simulink model "ModeInputHandle"  (R2018b)
settings: Solver=FixedStepDiscrete  StartTime=0.0  StopTime=10.0  FixedStep=0.01  RelTol=1e-3
undefined symbols (not defined in the file or in its folder): c, CmprtMdHMIReqExt2Tp1, CmprtMdHMIReqExtTp1, CmprtMdHMIReqTp1, d, e, EZESwReq1, f, g, IfVeSMSeStNumConfig, j, KeSMSuButtonLongPressedThrshldTm_Val, KeSMSuFoldType_Val, KeSMSwSeatSMSSeatMdTrigGapTimer_Val, KeSMSwSeatTrigWaitTimer_Val, KeSMSwSRSActiveValidTm_Val, LckUlckActvtFunc1, LstLckFunc1, LugSelectSw1, MdReqTp1, PowerMode1, SeatOccupiedSts1, SRSMode1, StPassCmprtMdCtrl_Md10_VCUConfig_Val, StPassCmprtMdCtrl_Md11_VCUConfig_Val, StPassCmprtMdCtrl_Md12_VCUConfig_Val, StPassCmprtMdCtrl_Md13_VCUConfig_Val, StPassCmprtMdCtrl_Md1_VCUConfig_Val, StPassCmprtMdCtrl_Md27_VCUConfig_Val, StPassCmprtMdCtrl_Md28_VCUConfig_Val, StPassCmprtMdCtrl_Md29_VCUConfig_Val, StPassCmprtMdCtrl_Md2_VCUConfig_Val, StPassCmprtMdCtrl_Md30_VCUConfig_Val, StPassCmprtMdCtrl_Md31_VCUConfig_Val, StPassCmprtMdCtrl_Md32_VCUConfig_Val, StPassCmprtMdCtrl_Md3_VCUConfig_Val, StPassCmprtMdCtrl_Md53_VCUConfig_Val, StPassCmprtMdCtrl_Md56_VCUConfig_Val, StPassCmprtMdCtrl_Md57_VCUConfig_Val, StPassCmprtMdCtrl_Md58_VCUConfig_Val, StPassCmprtMdCtrl_Md61_VCUConfig_Val, StPassCmprtMdCtrl_Md62_VCUConfig_Val, StPassCmprtMdCtrl_Md8_VCUConfig_Val, StPassCmprtMdCtrl_Md9_VCUConfig_Val, StSrv_StMd10_Config_Val, StSrv_StMd11_Config_Val, StSrv_StMd12_Config_Val, StSrv_StMd13_Config_Val, StSrv_StMd1_Config_Val, StSrv_StMd27_Config_Val, StSrv_StMd28_Config_Val, StSrv_StMd29_Config_Val, StSrv_StMd2_Config_Val, StSrv_StMd30_Config_Val, StSrv_StMd31_Config_Val, StSrv_StMd32_Config_Val, StSrv_StMd3_Config_Val, StSrv_StMd8_Config_Val, StSrv_StMd9_Config_Val, VehMovState1
libraries: MSMLib x91
(part 3 of 9)

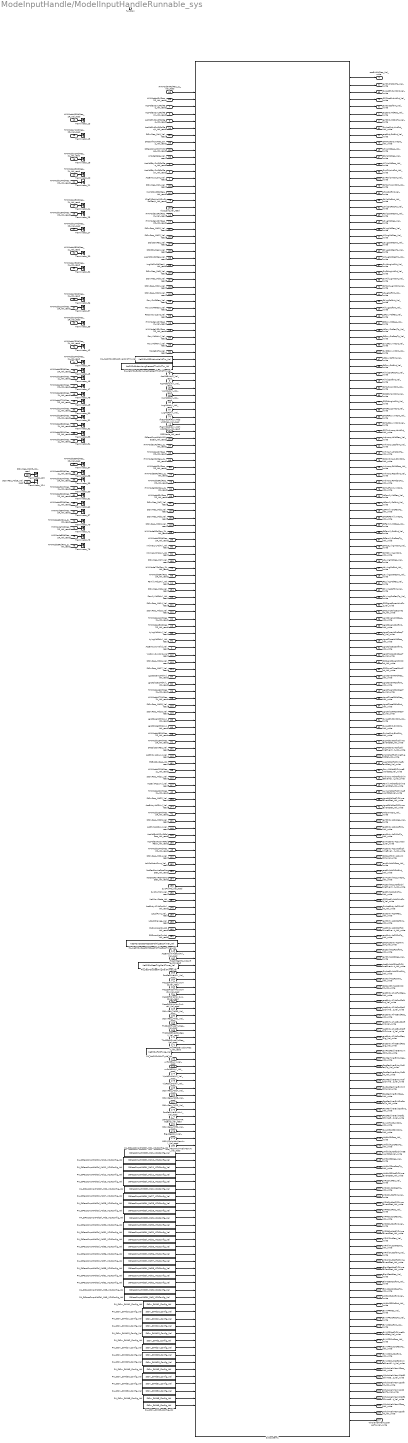
== system ModeInputHandle/ModelInputHandleRunnable_sys ==
  AcsEntry2LSwt_Val_read : Inport
  AcsEntrySwValid_Val_read : Inport  Port=2
  AcsMdEntyAvl_Val_read : Inport  Port=3
  AcsMdEtrySwRtRclReq_Val_read : Inport  Port=4
  AcsMdEtrySwRtRclReqV_Val_read : Inport  Port=5
  AcsMdExtAvl_Val_read : Inport  Port=6
  AcsMdExtSwLtRclReq_Val_read : Inport  Port=7
  AcsMdExtSwLtRclReqV_Val_read : Inport  Port=8
  AcsMdExtSwRtRclReq_Val_read : Inport  Port=9
  AcsMdExtSwRtRclReqV_Val_read : Inport  Port=10
  FamilyMdLtAvl_Val_read : Inport  Port=11
  FamilyMdRtAvl_Val_read : Inport  Port=12
  HMIMode10RclReq_2R_Val_read : Inport  Port=13
  HMIMode10RclReq_2L_Val_read : Inport  Port=14
  HMIMode11RclReq_2R_Val_read : Inport  Port=15
  HMIMode11RclReq_2L_Val_read : Inport  Port=16
  HMIMode12RclReq_2R_Val_read : Inport  Port=17
  HMIMode12RclReq_2L_Val_read : Inport  Port=18
  HMIMode13RclReq_2R_Val_read : Inport  Port=19
  HMIMode13RclReq_2L_Val_read : Inport  Port=20
  HMIMode14RclReq_2R_Val_read : Inport  Port=21
  HMIMode14RclReq_2L_Val_read : Inport  Port=22
  HMIMode15RclReq_2R_Val_read : Inport  Port=23
  HMIMode15RclReq_2L_Val_read : Inport  Port=24
  HMIMode16RclReq_2R_Val_read : Inport  Port=25
  HMIMode16RclReq_2L_Val_read : Inport  Port=26
  HMIMode17RclReq_2R_Val_read : Inport  Port=27
  HMIMode17RclReq_2L_Val_read : Inport  Port=28
  HMIMode18RclReq_2R_Val_read : Inport  Port=29
  HMIMode18RclReq_2L_Val_read : Inport  Port=30
  HMIMode19RclReq_2R_Val_read : Inport  Port=31
  HMIMode19RclReq_2L_Val_read : Inport  Port=32
  HMIMode1RclReq_2R_Val_read : Inport  Port=33
  HMIMode1RclReq_2L_Val_read : Inport  Port=34
  HMIMode20RclReq_2R_Val_read : Inport  Port=35
  HMIMode20RclReq_2L_Val_read : Inport  Port=36
  HMIMode21RclReq_2R_Val_read : Inport  Port=37
  HMIMode21RclReq_2L_Val_read : Inport  Port=38
  HMIMode22RclReq_2R_Val_read : Inport  Port=39
  HMIMode22RclReq_2L_Val_read : Inport  Port=40
  HMIMode23RclReq_2R_Val_read : Inport  Port=41
  HMIMode23RclReq_2L_Val_read : Inport  Port=42
  HMIMode24RclReq_2R_Val_read : Inport  Port=43
  HMIMode24RclReq_2L_Val_read : Inport  Port=44
  HMIMode25RclReq_2R_Val_read : Inport  Port=45
  HMIMode25RclReq_2L_Val_read : Inport  Port=46
  HMIMode26RclReq_2R_Val_read : Inport  Port=47
  HMIMode26RclReq_2L_Val_read : Inport  Port=48
  HMIMode27RclReq_2R_Val_read : Inport  Port=49
  HMIMode27RclReq_2L_Val_read : Inport  Port=50
  HMIMode28RclReq_2R_Val_read : Inport  Port=51
  HMIMode28RclReq_2L_Val_read : Inport  Port=52
  HMIMode29RclReq_2R_Val_read : Inport  Port=53
  HMIMode29RclReq_2L_Val_read : Inport  Port=54
  HMIMode2RclReq_2R_Val_read : Inport  Port=55
  HMIMode2RclReq_2L_Val_read : Inport  Port=56
  HMIMode30RclReq_2R_Val_read : Inport  Port=57
  HMIMode30RclReq_2L_Val_read : Inport  Port=58
  HMIMode31RclReq_2R_Val_read : Inport  Port=59
  HMIMode31RclReq_2L_Val_read : Inport  Port=60
  HMIMode32RclReq_2R_Val_read : Inport  Port=61
  HMIMode32RclReq_2L_Val_read : Inport  Port=62
  HMIMode3RclReq_2R_Val_read : Inport  Port=63
  HMIMode3RclReq_2L_Val_read : Inport  Port=64
  HMIMode4RclReq_2R_Val_read : Inport  Port=65
  HMIMode4RclReq_2L_Val_read : Inport  Port=66
  HMIMode5RclReq_2R_Val_read : Inport  Port=67
  HMIMode5RclReq_2L_Val_read : Inport  Port=68
  HMIMode6RclReq_2R_Val_read : Inport  Port=69
  HMIMode6RclReq_2L_Val_read : Inport  Port=70
  HMIMode7RclReq_2R_Val_read : Inport  Port=71
  HMIMode7RclReq_2L_Val_read : Inport  Port=72
  HMIMode8RclReq_2R_Val_read : Inport  Port=73
  HMIMode8RclReq_2L_Val_read : Inport  Port=74
  HMIMode9RclReq_2R_Val_read : Inport  Port=75
  HMIMode9RclReq_2L_Val_read : Inport  Port=76
  IfVeSMSbRrRcvyMdSwRclReq_Val_read : Inport  Port=77
  IfVeSMSbRrRcvyMdSwRclReqV_Val_read : Inport  Port=78
  IfVeSMSeVipMdSwRtRclReqV_Val_read : Inport  Port=79
  IntimacyLMdAvl_Val_read : Inport  Port=80
  IntimacyRMdAvl_Val_read : Inport  Port=81
  LgrstCloseLtMdAvl_Val_read : Inport  Port=82
  LgrstCloseRtMdAvl_Val_read : Inport  Port=83
  LgrstOpenLtMdAvl_Val_read : Inport  Port=84
  LgrstOpenRtMdAvl_Val_read : Inport  Port=85
  LugMdLtAvl_Val_read : Inport  Port=86
  LugMdRtAvl_Val_read : Inport  Port=87
  LugMdSwRclReq_Val_read : Inport  Port=88
  LugMdSwRclReqV_Val_read : Inport  Port=89
  LyingMdLtAvl_Val_read : Inport  Port=90
  LyingMdRtAvl_Val_read : Inport  Port=91
  ModeSrcTp_Val_read : Inport  Port=92
  oModeState_Val_read : Inport  Port=93
  RcvyMdLtAvl_Val_read : Inport  Port=94
  RcvyMdRtAvl_Val_read : Inport  Port=95
  RcvySwRtReq_Val_read : Inport  Port=96
  RcvySwRtReqV_Val_read : Inport  Port=97
  Recovery2LSwt_Val_read : Inport  Port=98
  SRSCnfmSwReq_67_2_Val_read : Inport  Port=99
  SRSMode_Val_read : Inport  Port=100
  SRSSlctSwReq_Val_read : Inport  Port=101
  StPassCmprtMdHMIReq_Val_read : Inport  Port=102
  StPassCmprtMdHMIReqExt_Val_read : Inport  Port=103
  StSlctSwReq_Val_read : Inport  Port=104
  StSlctSwReqV_Val_read : Inport  Port=105
  StSrvReq_Md1_Val_read : Inport  Port=106
  StSrvReq_Md10_Val_read : Inport  Port=107
  StSrvReq_Md11_Val_read : Inport  Port=108
  StSrvReq_Md12_Val_read : Inport  Port=109
  StSrvReq_Md13_Val_read : Inport  Port=110
  StSrvReq_Md14_Val_read : Inport  Port=111
  StSrvReq_Md15_Val_read : Inport  Port=112
  StSrvReq_Md16_Val_read : Inport  Port=113
  StSrvReq_Md17_Val_read : Inport  Port=114
  StSrvReq_Md18_Val_read : Inport  Port=115
  StSrvReq_Md19_Val_read : Inport  Port=116
  StSrvReq_Md2_Val_read : Inport  Port=117
  StSrvReq_Md20_Val_read : Inport  Port=118
  StSrvReq_Md21_Val_read : Inport  Port=119
  StSrvReq_Md22_Val_read : Inport  Port=120
  StSrvReq_Md23_Val_read : Inport  Port=121
  StSrvReq_Md24_Val_read : Inport  Port=122
  StSrvReq_Md25_Val_read : Inport  Port=123
  StSrvReq_Md26_Val_read : Inport  Port=124
  StSrvReq_Md27_Val_read : Inport  Port=125
  StSrvReq_Md28_Val_read : Inport  Port=126
  StSrvReq_Md29_Val_read : Inport  Port=127
  StSrvReq_Md3_Val_read : Inport  Port=128
  StSrvReq_Md30_Val_read : Inport  Port=129
  StSrvReq_Md31_Val_read : Inport  Port=130
  StSrvReq_Md32_Val_read : Inport  Port=131
  StSrvReq_Md4_Val_read : Inport  Port=132
  StSrvReq_Md5_Val_read : Inport  Port=133
  StSrvReq_Md6_Val_read : Inport  Port=134
  StSrvReq_Md7_Val_read : Inport  Port=135
  StSrvReq_Md8_Val_read : Inport  Port=136
  StSrvReq_Md9_Val_read : Inport  Port=137
  Vip2LSwt_Val_read : Inport  Port=138
  VipMdLtAvl_Val_read : Inport  Port=139
  VipMdRtAvl_Val_read : Inport  Port=140
  VipMdSwRtRclReq_Val_read : Inport  Port=141
  VipRcvySwValid_Val_read : Inport  Port=142
  AcsEntry4s2LAvl_Val_read : Inport  Port=143
  AcsEntry4s2RAvl_Val_read : Inport  Port=144
  AcsEntryAll4sBwdAvl_Val_read : Inport  Port=145
  AcsEntryAll4sFwdAvl_Val_read : Inport  Port=146
  AcsExit4s2LAvl_Val_read : Inport  Port=147
  AcsExit4s2RAvl_Val_read : Inport  Port=148
  AcsMdExt4SSwRtRclReq_Val_read : Inport  Port=149
  AcsMdExt4SSwRtRclReqV_Val_read : Inport  Port=150
  EZE4SSwReq_Val_read : Inport  Port=151
  LckUlckActvtFunc_Val_read : Inport  Port=152
  NotSecRowLeSeaOccStat_Val_read : Inport  Port=153
  NotSecRowRtSeaOccStat_Val_read : Inport  Port=154
  SysPwrMd_Val_read : Inport  Port=155
  SysPwrMdV_Val_read : Inport  Port=156
  VehMovState_Val_read : Inport  Port=157
  LstLckChange_Val_read : Inport  Port=158
  LstLckFunc_Val_read : Inport  Port=159
  RLDoorAjarSwAct_Val_read : Inport  Port=160
  RRDoorAjarSwAct_Val_read : Inport  Port=161
  IfVeSMSeStNumConfig_Val_read : Inport  Port=162
  PasReclinerAvl_Val_read : Inport  Port=163
  PassStFldDnMovSwAct_Val_read : Inport  Port=164
  PassStFldDnMovSwActV_Val_read : Inport  Port=165
  PassStFldUpMovSwAct_Val_read : Inport  Port=166
  PassStFldUpMovSwActV_Val_read : Inport  Port=167
  ThdRLtStExpdSwReq_Val_read : Inport  Port=168
  ThdRLtStExpdSwReqV_Val_read : Inport  Port=169
  ThdRRtStExpdSwReq_Val_read : Inport  Port=170
  ThdRRtStExpdSwReqV_Val_read : Inport  Port=171
  unfold3LAvl_Val_read : Inport  Port=172
  unfold3RAvl_Val_read : Inport  Port=173
  VipLtOutMdAvl_Val_read : Inport  Port=174
  VipRtOutMdAvl_Val_read : Inport  Port=175
  PasReclinerExitAvl_Val_read : Inport  Port=176
  StPassCmprtMdHMIReqExt2_Val_read : Inport  Port=177
  Big4SeatAvl_Val_read : Inport  Port=178
  M61WholeVehMemAvl_Val_read : Inport  Port=179
  M62WholeVehMemAvl_Val_read : Inport  Port=180
  function : TriggerPort  TriggerType=function-call  VariantControl=(inherit)  SampleTimeType=periodic  SampleTime=-1
  PA_KeSMSuButtonLongPressedThrshldTm_Val : Constant  Value=KeSMSuButtonLongPressedThrshldTm_Val
  PA_KeSMSuFoldType_Val : Constant  Value=KeSMSuFoldType_Val
  PA_KeSMSwSRSActiveValidTm_Val : Constant  Value=KeSMSwSRSActiveValidTm_Val
  PA_KeSMSwSeatSMSSeatMdTrigGapTimer_Val : Constant  Value=KeSMSwSeatSMSSeatMdTrigGapTimer_Val
  PA_KeSMSwSeatTrigWaitTimer_Val : Constant  Value=KeSMSwSeatTrigWaitTimer_Val
  PA_StPassCmprtMdCtrl_Md10_VCUConfig_Val : Constant  Value=StPassCmprtMdCtrl_Md10_VCUConfig_Val
  PA_StPassCmprtMdCtrl_Md11_VCUConfig_Val : Constant  Value=StPassCmprtMdCtrl_Md11_VCUConfig_Val
  PA_StPassCmprtMdCtrl_Md12_VCUConfig_Val : Constant  Value=StPassCmprtMdCtrl_Md12_VCUConfig_Val
  PA_StPassCmprtMdCtrl_Md13_VCUConfig_Val : Constant  Value=StPassCmprtMdCtrl_Md13_VCUConfig_Val
  PA_StPassCmprtMdCtrl_Md1_VCUConfig_Val : Constant  Value=StPassCmprtMdCtrl_Md1_VCUConfig_Val
  PA_StPassCmprtMdCtrl_Md27_VCUConfig_Val : Constant  Value=StPassCmprtMdCtrl_Md27_VCUConfig_Val
  PA_StPassCmprtMdCtrl_Md28_VCUConfig_Val : Constant  Value=StPassCmprtMdCtrl_Md28_VCUConfig_Val
  PA_StPassCmprtMdCtrl_Md29_VCUConfig_Val : Constant  Value=StPassCmprtMdCtrl_Md29_VCUConfig_Val
  PA_StPassCmprtMdCtrl_Md2_VCUConfig_Val : Constant  Value=StPassCmprtMdCtrl_Md2_VCUConfig_Val
  PA_StPassCmprtMdCtrl_Md30_VCUConfig_Val : Constant  Value=StPassCmprtMdCtrl_Md30_VCUConfig_Val
  PA_StPassCmprtMdCtrl_Md31_VCUConfig_Val : Constant  Value=StPassCmprtMdCtrl_Md31_VCUConfig_Val
  PA_StPassCmprtMdCtrl_Md32_VCUConfig_Val : Constant  Value=StPassCmprtMdCtrl_Md32_VCUConfig_Val
  PA_StPassCmprtMdCtrl_Md3_VCUConfig_Val : Constant  Value=StPassCmprtMdCtrl_Md3_VCUConfig_Val
  PA_StPassCmprtMdCtrl_Md53_VCUConfig_Val : Constant  Value=StPassCmprtMdCtrl_Md53_VCUConfig_Val
  PA_StPassCmprtMdCtrl_Md56_VCUConfig_Val : Constant  Value=StPassCmprtMdCtrl_Md56_VCUConfig_Val
  PA_StPassCmprtMdCtrl_Md57_VCUConfig_Val : Constant  Value=StPassCmprtMdCtrl_Md57_VCUConfig_Val
  PA_StPassCmprtMdCtrl_Md58_VCUConfig_Val : Constant  Value=StPassCmprtMdCtrl_Md58_VCUConfig_Val
  PA_StPassCmprtMdCtrl_Md61_VCUConfig_Val : Constant  Value=StPassCmprtMdCtrl_Md61_VCUConfig_Val
  PA_StPassCmprtMdCtrl_Md62_VCUConfig_Val : Constant  Value=StPassCmprtMdCtrl_Md62_VCUConfig_Val
  PA_StPassCmprtMdCtrl_Md8_VCUConfig_Val : Constant  Value=StPassCmprtMdCtrl_Md8_VCUConfig_Val
  PA_StPassCmprtMdCtrl_Md9_VCUConfig_Val : Constant  Value=StPassCmprtMdCtrl_Md9_VCUConfig_Val
  PA_StSrv_StMd10_Config_Val : Constant  Value=StSrv_StMd10_Config_Val
  PA_StSrv_StMd11_Config_Val : Constant  Value=StSrv_StMd11_Config_Val
  PA_StSrv_StMd12_Config_Val : Constant  Value=StSrv_StMd12_Config_Val
  PA_StSrv_StMd13_Config_Val : Constant  Value=StSrv_StMd13_Config_Val
  PA_StSrv_StMd1_Config_Val : Constant  Value=StSrv_StMd1_Config_Val
  PA_StSrv_StMd27_Config_Val : Constant  Value=StSrv_StMd27_Config_Val
  PA_StSrv_StMd28_Config_Val : Constant  Value=StSrv_StMd28_Config_Val
  PA_StSrv_StMd29_Config_Val : Constant  Value=StSrv_StMd29_Config_Val
  PA_StSrv_StMd2_Config_Val : Constant  Value=StSrv_StMd2_Config_Val
  PA_StSrv_StMd30_Config_Val : Constant  Value=StSrv_StMd30_Config_Val
  PA_StSrv_StMd31_Config_Val : Constant  Value=StSrv_StMd31_Config_Val
  PA_StSrv_StMd32_Config_Val : Constant  Value=StSrv_StMd32_Config_Val
  PA_StSrv_StMd3_Config_Val : Constant  Value=StSrv_StMd3_Config_Val
  PA_StSrv_StMd8_Config_Val : Constant  Value=StSrv_StMd8_Config_Val
  PA_StSrv_StMd9_Config_Val : Constant  Value=StSrv_StMd9_Config_Val
  Subsystem1 : Subsystem
  Terminator_{13,15,18,20..21,24..25,27,30,32,36..37,39,42,44..54,57..62,67,70..71,73,76,123..124} (38 alike) : Terminator
  acsEntyMdReq_Val_write : Outport
  acsEntyMdSrcTp_Val_write : Outport  Port=2
  acsEntySoftInt_Val_write : Outport  Port=3
  acsExtMdReq_Val_write : Outport  Port=4
  acsExtMdSrcTp_Val_write : Outport  Port=5
  acsExtSoftInt_Val_write : Outport  Port=6
  acsMdEntryNotf1ChimeEventStat_Val_write : Outport  Port=7
  acsMdExtNotf1ChimeEventStat_Val_write : Outport  Port=8
  AllLugMdReq_Val_write : Outport  Port=9
  AllLugSoftInt_Val_write : Outport  Port=10
  AllLugSrcReqTp_Val_write : Outport  Port=11
  AllVipMdReq_Val_write : Outport  Port=12
  AllVipSoftInt_Val_write : Outport  Port=13
  AllVipSrcReqTp_Val_write : Outport  Port=14
  FamilyMdNotf1ChimeEventStat_Val_write : Outport  Port=15
  IntimacyMdNotf1ChimeEventStat_Val_write : Outport  Port=16
  IntimacyLtMdReq_Val_write : Outport  Port=17
  IntimacyLtMdSrcTp_Val_write : Outport  Port=18
  IntimacyRtMdReq_Val_write : Outport  Port=19
  IntimacyRtMdSrcTp_Val_write : Outport  Port=20
  IntimacyRtSoftInt_Val_write : Outport  Port=21
  IntimacyLtSoftInt_Val_write : Outport  Port=22
  LtFamilyMdReq_Val_write : Outport  Port=23
  LtFamilySoftInt_Val_write : Outport  Port=24
  LtFamilySrcReqTp_Val_write : Outport  Port=25
  LtLyingMdReq_Val_write : Outport  Port=26
  LtLyingSoftInt_Val_write : Outport  Port=27
  LtLyingSrcReqTp_Val_write : Outport  Port=28
  LgrstCloseLtMdReq_Val_write : Outport  Port=29
  LgrstCloseLtSrcReqTp_Val_write : Outport  Port=30
  LgrstCloseLtSoftInt_Val_write : Outport  Port=31
  LgrstCloseRtMdReq_Val_write : Outport  Port=32
  LgrstCloseRtSrcReqTp_Val_write : Outport  Port=33
  LgrstCloseRtSoftInt_Val_write : Outport  Port=34
  LgrstLtMdNotf1ChimeEventStat_Val_write : Outport  Port=35
  LgrstOpenLtMdReq_Val_write : Outport  Port=36
  LgrstOpenLtSrcReqTp_Val_write : Outport  Port=37
  LgrstOpenLtSoftInt_Val_write : Outport  Port=38
  LgrstOpenRtMdReq_Val_write : Outport  Port=39
  LgrstOpenRtSrcReqTp_Val_write : Outport  Port=40
  LgrstOpenRtSoftInt_Val_write : Outport  Port=41
  LgrstRtMdNotf1ChimeEventStat_Val_write : Outport  Port=42
  LtLugMdReq_Val_write : Outport  Port=43
  LtLugSoftInt_Val_write : Outport  Port=44
  LtLugSrcReqTp_Val_write : Outport  Port=45
  LtRcvyMdReq_Val_write : Outport  Port=46
  LtRcvySoftInt_Val_write : Outport  Port=47
  LtRcvySrcReqTp_Val_write : Outport  Port=48
  LtVipMdReq_Val_write : Outport  Port=49
  LtVipSoftInt_Val_write : Outport  Port=50
  LtVipSrcReqTp_Val_write : Outport  Port=51
  LugMdNotf1ChimeEventStat_Val_write : Outport  Port=52
  LyingMdNotf1ChimeEventStat_Val_write : Outport  Port=53
  RcvyMdNotf1ChimeEventStat_Val_write : Outport  Port=54
  RtFamilyMdReq_Val_write : Outport  Port=55
  RtFamilySoftInt_Val_write : Outport  Port=56
  RtFamilySrcReqTp_Val_write : Outport  Port=57
  RtLugMdReq_Val_write : Outport  Port=58
  RtLugSoftInt_Val_write : Outport  Port=59
  RtLugSrcReqTp_Val_write : Outport  Port=60
  RtLyingMdReq_Val_write : Outport  Port=61
  RtLyingSoftInt_Val_write : Outport  Port=62
  RtLyingSrcReqTp_Val_write : Outport  Port=63
  RtRcvyMdReq_Val_write : Outport  Port=64
  RtRcvySoftInt_Val_write : Outport  Port=65
  RtRcvySrcReqTp_Val_write : Outport  Port=66
  RtVipMdReq_Val_write : Outport  Port=67
  RtVipSoftInt_Val_write : Outport  Port=68
  RtVipSrcReqTp_Val_write : Outport  Port=69
  SRSAcsEntyIntCnt_Val_write : Outport  Port=70
  SRSAcsExtIntCnt_Val_write : Outport  Port=71
  SRSAllLugIntCnt_Val_write : Outport  Port=72
  SRSAllVipIntCnt_Val_write : Outport  Port=73
  SRSIntimacyLtIntCnt_Val_write : Outport  Port=74
  SRSIntimacyRtIntCnt_Val_write : Outport  Port=75
  SRSLtFamilyIntCnt_Val_write : Outport  Port=76
  SRSLtLugIntCnt_Val_write : Outport  Port=77
  SRSLtLyingIntCnt_Val_write : Outport  Port=78
  SRSLtRcvyIntCnt_Val_write : Outport  Port=79
  SRSLtVipIntCnt_Val_write : Outport  Port=80
  SRSLgrstCloseLtIntCnt_Val_write : Outport  Port=81
  SRSLgrstCloseRtIntCnt_Val_write : Outport  Port=82
  SRSLgrstOpenLtIntCnt_Val_write : Outport  Port=83
  SRSLgrstOpenRtIntCnt_Val_write : Outport  Port=84
  SRSRtFamilyIntCnt_Val_write : Outport  Port=85
  SRSRtLugIntCnt_Val_write : Outport  Port=86
  SRSRtLyingIntCnt_Val_write : Outport  Port=87
  SRSRtRcvyIntCnt_Val_write : Outport  Port=88
  SRSRtVipIntCnt_Val_write : Outport  Port=89
  SwAcsEntyBIntCnt_Val_write : Outport  Port=90
  SwAcsEntyLIntCnt_Val_write : Outport  Port=91
  SwAcsEntyRIntCnt_Val_write : Outport  Port=92
  SwAcsExtLIntCnt_Val_write : Outport  Port=93
  SwAcsExtRIntCnt_Val_write : Outport  Port=94
  SwAllLugIntCnt_Val_write : Outport  Port=95
  SwLfVipIntCnt_Val_write : Outport  Port=96
  SwLtLugIntCnt_Val_write : Outport  Port=97
  SwLtRcvyIntCnt_Val_write : Outport  Port=98
  SwRtLugIntCnt_Val_write : Outport  Port=99
  SwRtRcvyIntCnt_Val_write : Outport  Port=100
  SwRtVipIntCnt_Val_write : Outport  Port=101
  VipMdNotf1ChimeEventStat_Val_write : Outport  Port=102
  MdSWIntSrc_Val_write : Outport  Port=103
  SwAcsEntry4s2LIntCnt_Val_write : Outport  Port=104
  AcsEntry4s2LNotf1ChimeEventStat_Val_write : Outport  Port=105
  acsEntry4s2LReq_Val_write : Outport  Port=106
  acsEntry4s2LSoftInt_Val_write : Outport  Port=107
  acsEntry4s2LSrcTp_Val_write : Outport  Port=108
  SwAcsEntry4s2RIntCnt_Val_write : Outport  Port=109
  AcsEntry4s2RNotf1ChimeEventStat_Val_write : Outport  Port=110
  acsEntry4s2RReq_Val_write : Outport  Port=111
  acsEntry4s2RSoftInt_Val_write : Outport  Port=112
  acsEntry4s2RSrcTp_Val_write : Outport  Port=113
  AcsEntryAll4sBwdNotf1ChimeEventStat_Val_write : Outport  Port=114
  AcsEntryAll4sFwdNotf1ChimeEventStat_Val_write : Outport  Port=115
  SwAcsExit4s2LIntCnt_Val_write : Outport  Port=116
  AcsExit4s2LNotf1ChimeEventStat_Val_write : Outport  Port=117
  acsExit4s2LReq_Val_write : Outport  Port=118
  acsExit4s2LSoftInt_Val_write : Outport  Port=119
  acsExit4s2LSrcTp_Val_write : Outport  Port=120
  SwAcsExit4s2RIntCnt_Val_write : Outport  Port=121
  AcsExit4s2RNotf1ChimeEventStat_Val_write : Outport  Port=122
  acsExit4s2RReq_Val_write : Outport  Port=123
  acsExit4s2RSoftInt_Val_write : Outport  Port=124
  acsExit4s2RSrcTp_Val_write : Outport  Port=125
  SRSAcsEntry4s2LIntCnt_Val_write : Outport  Port=126
  SRSAcsEntry4s2RIntCnt_Val_write : Outport  Port=127
  SRSAcsExit4s2LIntCnt_Val_write : Outport  Port=128
  SRSAcsExit4s2RIntCnt_Val_write : Outport  Port=129
  acsEntryAll4sBwdReq_Val_write : Outport  Port=130
  acsEntryAll4sBwdSoftInt_Val_write : Outport  Port=131
  acsEntryAll4sFwdReq_Val_write : Outport  Port=132
  acsEntryAll4sFwdSoftInt_Val_write : Outport  Port=133
  acsEntryAll4sBwdReqSig_Val_write : Outport  Port=134
  acsEntryAll4sFwdReqSig_Val_write : Outport  Port=135
  PasReclinerEntryNotf1ChimeEventStat_Val_write : Outport  Port=136
  PasReclinerEntryReq_Val_write : Outport  Port=137
  PasReclinerEntrySoftInt_Val_write : Outport  Port=138
  PasReclinerEntrySrcReqTp_Val_write : Outport  Port=139
  PasReclinerExitNotf1ChimeEventStat_Val_write : Outport  Port=140
  PasReclinerExitReq_Val_write : Outport  Port=141
  PasReclinerExitSoftInt_Val_write : Outport  Port=142
  PasReclinerExitSrcReqTp_Val_write : Outport  Port=143
  Unfold3LNotf1ChimeEventStat_Val_write : Outport  Port=144
  Unfold3LReq_Val_write : Outport  Port=145
  Unfold3LsrcReqTp_Val_write : Outport  Port=146
  Unfold3RNotf1ChimeEventStat_Val_write : Outport  Port=147
  Unfold3RReq_Val_write : Outport  Port=148
  Unfold3RsrcReqTp_Val_write : Outport  Port=149
  VIPAllOutNotf1ChimeEventStat_Val_write : Outport  Port=150
  VIPAllOutReq_Val_write : Outport  Port=151
  VIPAllOutSoftInt_Val_write : Outport  Port=152
  VIPAllOutsrcReqTp_Val_write : Outport  Port=153
  VIPLtOutNotf1ChimeEventStat_Val_write : Outport  Port=154
  VIPLtOutReq_Val_write : Outport  Port=155
  VIPLtOutSoftInt_Val_write : Outport  Port=156
  VIPLtOutsrcReqTp_Val_write : Outport  Port=157
  VIPRtOutNotf1ChimeEventStat_Val_write : Outport  Port=158
  VIPRtOutReq_Val_write : Outport  Port=159
  VIPRtOutSoftInt_Val_write : Outport  Port=160
  VIPRtOutsrcReqTp_Val_write : Outport  Port=161
  SwPasReclinerEntryIntCnt_Val_write : Outport  Port=162
  SwPasReclinerExitIntCnt_Val_write : Outport  Port=163
  SwUnfold3LIntCnt_Val_write : Outport  Port=164
  SwUnfold3RIntCnt_Val_write : Outport  Port=165
  Big4SeatNotf1ChimeEventStat_Val_write : Outport  Port=166
  Big4SeatReq_Val_write : Outport  Port=167
  Big4SeatSoftInt_Val_write : Outport  Port=168
  Big4SeatsrcReqTp_Val_write : Outport  Port=169
  Unfold3LSoftInt_Val_write : Outport  Port=170
  Unfold3RSoftInt_Val_write : Outport  Port=171
  ExVIPRNotf1ChimeEventStat_Val_write : Outport  Port=172
  ExVIPROutNotf1ChimeEventStat_Val_write : Outport  Port=173
  ExVIPROutReq_Val_write : Outport  Port=174
  ExVIPROutSoftInt_Val_write : Outport  Port=175
  ExVIPROutsrcReqTp_Val_write : Outport  Port=176
  ExVIPRReq_Val_write : Outport  Port=177
  ExVIPRSoftInt_Val_write : Outport  Port=178
  ExVIPRsrcReqTp_Val_write : Outport  Port=179
  WholeVehMem1Notf1ChimeEventStat_Val_write : Outport  Port=180
  WholeVehMem1Req_Val_write : Outport  Port=181
  WholeVehMem1SoftInt_Val_write : Outport  Port=182
  WholeVehMem1srcReqTp_Val_write : Outport  Port=183
  WholeVehMem2Notf1ChimeEventStat_Val_write : Outport  Port=184
  WholeVehMem2Req_Val_write : Outport  Port=185
  WholeVehMem2SoftInt_Val_write : Outport  Port=186
  WholeVehMem2srcReqTp_Val_write : Outport  Port=187
  wires:
  HMIMode10RclReq_2R_Val_read/1 -> Terminator_13/1
  HMIMode11RclReq_2R_Val_read/1 -> Terminator_15/1
  HMIMode12RclReq_2L_Val_read/1 -> Terminator_18/1
  HMIMode13RclReq_2L_Val_read/1 -> Terminator_20/1
  HMIMode14RclReq_2R_Val_read/1 -> Terminator_21/1
  HMIMode15RclReq_2L_Val_read/1 -> Terminator_24/1
  HMIMode16RclReq_2R_Val_read/1 -> Terminator_25/1
  HMIMode17RclReq_2R_Val_read/1 -> Terminator_27/1
  HMIMode18RclReq_2L_Val_read/1 -> Terminator_30/1
  HMIMode19RclReq_2L_Val_read/1 -> Terminator_32/1
  HMIMode20RclReq_2L_Val_read/1 -> Terminator_36/1
  HMIMode21RclReq_2R_Val_read/1 -> Terminator_37/1
  HMIMode22RclReq_2R_Val_read/1 -> Terminator_39/1
  HMIMode23RclReq_2L_Val_read/1 -> Terminator_42/1
  HMIMode24RclReq_2L_Val_read/1 -> Terminator_44/1
  HMIMode25RclReq_2R_Val_read/1 -> Terminator_45/1
  HMIMode25RclReq_2L_Val_read/1 -> Terminator_46/1
  HMIMode26RclReq_2R_Val_read/1 -> Terminator_47/1
  HMIMode26RclReq_2L_Val_read/1 -> Terminator_48/1
  HMIMode27RclReq_2R_Val_read/1 -> Terminator_49/1
  HMIMode27RclReq_2L_Val_read/1 -> Terminator_50/1
  HMIMode28RclReq_2R_Val_read/1 -> Terminator_51/1
  HMIMode28RclReq_2L_Val_read/1 -> Terminator_52/1
  HMIMode29RclReq_2R_Val_read/1 -> Terminator_53/1
  HMIMode29RclReq_2L_Val_read/1 -> Terminator_54/1
  HMIMode30RclReq_2R_Val_read/1 -> Terminator_57/1
  HMIMode30RclReq_2L_Val_read/1 -> Terminator_58/1
  HMIMode31RclReq_2R_Val_read/1 -> Terminator_59/1
  HMIMode31RclReq_2L_Val_read/1 -> Terminator_60/1
  HMIMode32RclReq_2R_Val_read/1 -> Terminator_61/1
  HMIMode32RclReq_2L_Val_read/1 -> Terminator_62/1
  HMIMode5RclReq_2R_Val_read/1 -> Terminator_67/1
  HMIMode6RclReq_2L_Val_read/1 -> Terminator_70/1
  HMIMode7RclReq_2R_Val_read/1 -> Terminator_71/1
  HMIMode8RclReq_2R_Val_read/1 -> Terminator_73/1
  HMIMode9RclReq_2L_Val_read/1 -> Terminator_76/1
  StSrvReq_Md25_Val_read/1 -> Terminator_123/1
  StSrvReq_Md26_Val_read/1 -> Terminator_124/1
  Subsystem1/95(VipMdNotf1ChimeEventStat) -> VipMdNotf1ChimeEventStat_Val_write/1
  Subsystem1/96(LugMdNotf1ChimeEventStat) -> LugMdNotf1ChimeEventStat_Val_write/1
  Subsystem1/100(LyingMdNotf1ChimeEventStat) -> LyingMdNotf1ChimeEventStat_Val_write/1
  Subsystem1/97(RcvyMdNotf1ChimeEventStat) -> RcvyMdNotf1ChimeEventStat_Val_write/1
  Subsystem1/98(IntimacyMdNotf1ChimeEventStat) -> IntimacyMdNotf1ChimeEventStat_Val_write/1
  Subsystem1/99(FamilyMdNotf1ChimeEventStat) -> FamilyMdNotf1ChimeEventStat_Val_write/1
  Subsystem1/101(LgrstLtMdNotf1ChimeEventStat) -> LgrstLtMdNotf1ChimeEventStat_Val_write/1
  Subsystem1/102(LgrstRtMdNotf1ChimeEventStat) -> LgrstRtMdNotf1ChimeEventStat_Val_write/1
  Subsystem1/93(acsMdExtNotf1ChimeEventStat) -> acsMdExtNotf1ChimeEventStat_Val_write/1
  Subsystem1/94(acsMdEntryNotf1ChimeEventStat) -> acsMdEntryNotf1ChimeEventStat_Val_write/1
  Subsystem1/91(SwAcsEntyRIntCnt) -> SwAcsEntyRIntCnt_Val_write/1
  Subsystem1/92(SwAcsEntyBIntCnt) -> SwAcsEntyBIntCnt_Val_write/1
  Subsystem1/8(SwAcsEntyLIntCnt) -> SwAcsEntyLIntCnt_Val_write/1
  Subsystem1/1(acsExtMdReq) -> acsExtMdReq_Val_write/1
  Subsystem1/2(acsExtMdSrcTp) -> acsExtMdSrcTp_Val_write/1
  Subsystem1/3(SwAcsExtLIntCnt) -> SwAcsExtLIntCnt_Val_write/1
  Subsystem1/90(SwAcsExtRIntCnt) -> SwAcsExtRIntCnt_Val_write/1
  Subsystem1/83(SRSLgrstCloseRtIntCnt) -> SRSLgrstCloseRtIntCnt_Val_write/1
  Subsystem1/82(SRSLgrstOpenRtIntCnt) -> SRSLgrstOpenRtIntCnt_Val_write/1
  Subsystem1/76(LgrstOpenLtMdReq) -> LgrstOpenLtMdReq_Val_write/1
  Subsystem1/87(LgrstCloseRtMdReq) -> LgrstCloseRtMdReq_Val_write/1
  Subsystem1/5(acsExtSoftInt) -> acsExtSoftInt_Val_write/1
  Subsystem1/4(SRSAcsExtIntCnt) -> SRSAcsExtIntCnt_Val_write/1
  Subsystem1/6(acsEntyMdReq) -> acsEntyMdReq_Val_write/1
  Subsystem1/7(acsEntyMdSrcTp) -> acsEntyMdSrcTp_Val_write/1
  Subsystem1/9(acsEntySoftInt) -> acsEntySoftInt_Val_write/1
  Subsystem1/23(AllLugMdReq) -> AllLugMdReq_Val_write/1
  Subsystem1/26(AllLugSrcReqTp) -> AllLugSrcReqTp_Val_write/1
  Subsystem1/33(AllLugSoftInt) -> AllLugSoftInt_Val_write/1
  Subsystem1/43(AllVipSoftInt) -> AllVipSoftInt_Val_write/1
  Subsystem1/42(AllVipSrcReqTp) -> AllVipSrcReqTp_Val_write/1
  Subsystem1/13(AllVipMdReq) -> AllVipMdReq_Val_write/1
  Subsystem1/51(IntimacyLtMdReq) -> IntimacyLtMdReq_Val_write/1
  Subsystem1/52(IntimacyLtSoftInt) -> IntimacyLtSoftInt_Val_write/1
  Subsystem1/53(IntimacyLtMdSrcTp) -> IntimacyLtMdSrcTp_Val_write/1
  Subsystem1/55(IntimacyRtMdReq) -> IntimacyRtMdReq_Val_write/1
  Subsystem1/56(IntimacyRtSoftInt) -> IntimacyRtSoftInt_Val_write/1
  Subsystem1/57(IntimacyRtMdSrcTp) -> IntimacyRtMdSrcTp_Val_write/1
  Subsystem1/75(SRSLgrstCloseLtIntCnt) -> SRSLgrstCloseLtIntCnt_Val_write/1
  Subsystem1/74(SRSLgrstOpenLtIntCnt) -> SRSLgrstOpenLtIntCnt_Val_write/1
  Subsystem1/10(SRSAcsEntyIntCnt) -> SRSAcsEntyIntCnt_Val_write/1
  Subsystem1/59(FamilyMdLtReq) -> LtFamilyMdReq_Val_write/1
  Subsystem1/60(FamilyLtSoftInt) -> LtFamilySoftInt_Val_write/1
  Subsystem1/61(FamilyLtSrcReqTp) -> LtFamilySrcReqTp_Val_write/1
  Subsystem1/68(LtLyingMdReq) -> LtLyingMdReq_Val_write/1
  Subsystem1/69(LtLyingSoftInt) -> LtLyingSoftInt_Val_write/1
  Subsystem1/70(LtLyingSrcReqTp) -> LtLyingSrcReqTp_Val_write/1
  Subsystem1/71(RtLyingMdReq) -> RtLyingMdReq_Val_write/1
  Subsystem1/72(RtLyingSoftInt) -> RtLyingSoftInt_Val_write/1
  Subsystem1/73(RtLyingSrcReqTp) -> RtLyingSrcReqTp_Val_write/1
  Subsystem1/63(FamilyMdRtReq) -> RtFamilyMdReq_Val_write/1
  Subsystem1/64(FamilyRtSoftInt) -> RtFamilySoftInt_Val_write/1
  Subsystem1/65(FamilyRtSrcReqTp) -> RtFamilySrcReqTp_Val_write/1
  Subsystem1/22(RtLugMdReq) -> RtLugMdReq_Val_write/1
  Subsystem1/32(RtLugSoftInt) -> RtLugSoftInt_Val_write/1
  Subsystem1/25(RtLugSrcReqTp) -> RtLugSrcReqTp_Val_write/1
  Subsystem1/21(LtLugMdReq) -> LtLugMdReq_Val_write/1
  Subsystem1/24(LtLugSrcReqTp) -> LtLugSrcReqTp_Val_write/1
  Subsystem1/31(LtLugSoftInt) -> LtLugSoftInt_Val_write/1
  Subsystem1/34(LtRcvyMdReq) -> LtRcvyMdReq_Val_write/1
  Subsystem1/40(LtRcvySoftInt) -> LtRcvySoftInt_Val_write/1
  Subsystem1/36(LtRcvySrcReqTp) -> LtRcvySrcReqTp_Val_write/1
  Subsystem1/11(LtVipMdReq) -> LtVipMdReq_Val_write/1
  Subsystem1/17(LtVipSoftInt) -> LtVipSoftInt_Val_write/1
  Subsystem1/19(LtVipSrcReqTp) -> LtVipSrcReqTp_Val_write/1
  Subsystem1/12(RtVipMdReq) -> RtVipMdReq_Val_write/1
  Subsystem1/18(RtVipSoftInt) -> RtVipSoftInt_Val_write/1
  Subsystem1/20(RtVipSrcReqTp) -> RtVipSrcReqTp_Val_write/1
  Subsystem1/35(RtRcvyMdReq) -> RtRcvyMdReq_Val_write/1
  Subsystem1/37(RtRcvySrcReqTp) -> RtRcvySrcReqTp_Val_write/1
  Subsystem1/41(RtRcvySoftInt) -> RtRcvySoftInt_Val_write/1
  Subsystem1/38(SwLtRcvyIntCnt) -> SwLtRcvyIntCnt_Val_write/1
  Subsystem1/39(SwRtRcvyIntCnt) -> SwRtRcvyIntCnt_Val_write/1
  Subsystem1/27(SwLtLugIntCnt) -> SwLtLugIntCnt_Val_write/1
  Subsystem1/28(SwRtLugIntCnt) -> SwRtLugIntCnt_Val_write/1
  Subsystem1/29(SwAllLugIntCnt) -> SwAllLugIntCnt_Val_write/1
  Subsystem1/49(SRSLtRcvyIntCnt) -> SRSLtRcvyIntCnt_Val_write/1
  Subsystem1/48(SRSRtRcvyIntCnt) -> SRSRtRcvyIntCnt_Val_write/1
  Subsystem1/66(SRSLtLyingIntCnt) -> SRSLtLyingIntCnt_Val_write/1
  Subsystem1/67(SRSRtLyingIntCnt) -> SRSRtLyingIntCnt_Val_write/1
  Subsystem1/62(SRSFamilyRtIntCnt) -> SRSRtFamilyIntCnt_Val_write/1
  Subsystem1/58(SRSFamilyLtIntCnt) -> SRSLtFamilyIntCnt_Val_write/1
  Subsystem1/54(SRSIntimacyRtIntCnt) -> SRSIntimacyRtIntCnt_Val_write/1
  Subsystem1/14(SwLfVipIntCnt) -> SwLfVipIntCnt_Val_write/1
  Subsystem1/15(SwRtVipIntCnt) -> SwRtVipIntCnt_Val_write/1
  Subsystem1/16(SRSAllVipIntCnt) -> SRSAllVipIntCnt_Val_write/1
  Subsystem1/30(SRSAllLugIntCnt) -> SRSAllLugIntCnt_Val_write/1
  Subsystem1/44(SRSLfVipIntCnt) -> SRSLtVipIntCnt_Val_write/1
  Subsystem1/45(SRSRtVipIntCnt) -> SRSRtVipIntCnt_Val_write/1
  Subsystem1/46(SRSLfLugIntCnt) -> SRSLtLugIntCnt_Val_write/1
  Subsystem1/47(SRSRtLugIntCnt) -> SRSRtLugIntCnt_Val_write/1
  Subsystem1/50(SRSIntimacyLtIntCnt) -> SRSIntimacyLtIntCnt_Val_write/1
  Subsystem1/78(LgrstOpenLtSrcReqTp) -> LgrstOpenLtSrcReqTp_Val_write/1
  Subsystem1/77(LgrstOpenLtSoftInt) -> LgrstOpenLtSoftInt_Val_write/1
  Subsystem1/79(LgrstCloseLtMdReq) -> LgrstCloseLtMdReq_Val_write/1
  Subsystem1/80(LgrstCloseLtSoftInt) -> LgrstCloseLtSoftInt_Val_write/1
  Subsystem1/81(LgrstCloseLtSrcReqTp) -> LgrstCloseLtSrcReqTp_Val_write/1
  Subsystem1/84(LgrstOpenRtMdReq) -> LgrstOpenRtMdReq_Val_write/1
  Subsystem1/85(LgrstOpenRtSoftInt) -> LgrstOpenRtSoftInt_Val_write/1
  Subsystem1/86(LgrstOpenRtSrcReqTp) -> LgrstOpenRtSrcReqTp_Val_write/1
  Subsystem1/88(LgrstCloseRtSoftInt) -> LgrstCloseRtSoftInt_Val_write/1
  Subsystem1/89(LgrstCloseRtSrcReqTp) -> LgrstCloseRtSrcReqTp_Val_write/1
  AcsEntry2LSwt_Val_read/1 -> Subsystem1/13(AcsEntry2LSwt)
  oModeState_Val_read/1 -> Subsystem1/10(modeAdjustReqDelay)
  HMIMode4RclReq_2L_Val_read/1 -> Subsystem1/1(AcsMdExtMdHMI2LRclReq)
  HMIMode4RclReq_2R_Val_read/1 -> Subsystem1/2(AcsMdExtMdHMI2RRclReq)
  AcsMdExtSwLtRclReq_Val_read/1 -> Subsystem1/3(AcsMdExtSwLtRclReq)
  AcsMdExtSwRtRclReq_Val_read/1 -> Subsystem1/5(AcsMdExtSwRtRclReq)
  AcsMdExtSwLtRclReqV_Val_read/1 -> Subsystem1/4(AcsMdExtSwLtRclReqV)
  AcsMdExtSwRtRclReqV_Val_read/1 -> Subsystem1/6(AcsMdExtSwRtRclReqV)
  StSrvReq_Md4_Val_read/1 -> Subsystem1/7(StPassAcsMdExtReq)
  SRSCnfmSwReq_67_2_Val_read/1 -> Subsystem1/8(SRSCnfmSwReq_67_2)
  StPassCmprtMdHMIReq_Val_read/1 -> Subsystem1/9(StPassCmprtMdHMIReq)
  AcsMdEtrySwRtRclReq_Val_read/1 -> Subsystem1/11(AcsMdEtrySwRtRclReq)
  AcsMdEtrySwRtRclReqV_Val_read/1 -> Subsystem1/12(AcsMdEtrySwRtRclReqV)
  StSrvReq_Md1_Val_read/1 -> Subsystem1/14(StPassAcsMdEtryReq)
  VipMdSwRtRclReq_Val_read/1 -> Subsystem1/15(VipMdSwRtRclReq)
  IfVeSMSeVipMdSwRtRclReqV_Val_read/1 -> Subsystem1/16(VipMdSwRtRclReqV)
  Vip2LSwt_Val_read/1 -> Subsystem1/17(Vip2LSwt)
  HMIMode10RclReq_2L_Val_read/1 -> Subsystem1/18(VIPMdHMI2LRclReq)
  HMIMode12RclReq_2R_Val_read/1 -> Subsystem1/19(VIPMdHMI2RRclReq)
  StSrvReq_Md10_Val_read/1 -> Subsystem1/20(StPassVipMdLtReq)
  StSrvReq_Md12_Val_read/1 -> Subsystem1/21(StPassVipMdRtReq)
  StSlctSwReq_Val_read/1 -> Subsystem1/22(StSlctSwReq)
  StSlctSwReqV_Val_read/1 -> Subsystem1/23(StSlctSwReqV)
  LugMdSwRclReq_Val_read/1 -> Subsystem1/24(LugMdSwRclReq)
  LugMdSwRclReqV_Val_read/1 -> Subsystem1/25(LugMdSwRclReqV)
  StSrvReq_Md8_Val_read/1 -> Subsystem1/26(StPassLugMdLtReq)
  StSrvReq_Md9_Val_read/1 -> Subsystem1/27(StPassLugMdRtReq)
  StSrvReq_Md11_Val_read/1 -> Subsystem1/28(StPassRcvyMdLtReq)
  StSrvReq_Md13_Val_read/1 -> Subsystem1/29(StPassRcvyMdRtReq)
  RcvySwRtReq_Val_read/1 -> Subsystem1/30(RcvySwRtReq)
  RcvySwRtReqV_Val_read/1 -> Subsystem1/31(RcvySwRtReqV)
  Recovery2LSwt_Val_read/1 -> Subsystem1/32(Recovery2LSwt)
  HMIMode11RclReq_2L_Val_read/1 -> Subsystem1/33(RcvyMdHMI2LRclReq)
  HMIMode13RclReq_2R_Val_read/1 -> Subsystem1/34(RcvyMdHMI2RRclReq)
  RcvyMdLtAvl_Val_read/1 -> Subsystem1/35(RcvyMdLtAvl)
  RcvyMdRtAvl_Val_read/1 -> Subsystem1/36(RcvyMdRtAvl)
  ModeSrcTp_Val_read/1 -> Subsystem1/37(ModeSrcTpLt)
  PA_KeSMSwSRSActiveValidTm_Val/1 -> Subsystem1/38(KeSMSwSRSActiveValidTm)
  PA_KeSMSuButtonLongPressedThrshldTm_Val/1 -> Subsystem1/39(KeSMSuButtonLongPressedThrshldTm)
  AcsMdExtAvl_Val_read/1 -> Subsystem1/40(AcsMdExtAvl)
  AcsMdEntyAvl_Val_read/1 -> Subsystem1/41(AcsMdEntyAvl)
  VipMdLtAvl_Val_read/1 -> Subsystem1/42(VipMdLtAvl)
  VipMdRtAvl_Val_read/1 -> Subsystem1/43(VipMdRtAvl)
  LugMdLtAvl_Val_read/1 -> Subsystem1/44(LugMdLtAvl)
  LugMdRtAvl_Val_read/1 -> Subsystem1/45(LugMdRtAvl)
  IfVeSMSbRrRcvyMdSwRclReq_Val_read/1 -> Subsystem1/46(RrRcvyMdSwRclReq)
  IfVeSMSbRrRcvyMdSwRclReqV_Val_read/1 -> Subsystem1/47(RrRcvyMdSwRclReqV)
  SRSMode_Val_read/1 -> Subsystem1/48(SRSMode)
  StPassCmprtMdHMIReqExt_Val_read/1 -> Subsystem1/49(StPassCmprtMdHMIReqExt)
  HMIMode1RclReq_2L_Val_read/1 -> Subsystem1/50(AcsMdEntyHMI2LRclReq)
  HMIMode1RclReq_2R_Val_read/1 -> Subsystem1/51(AcsMdEntyHMI2RRclReq)
  HMIMode2RclReq_2L_Val_read/1 -> Subsystem1/52(VIPAll2LHMIRclReq)
  HMIMode2RclReq_2R_Val_read/1 -> Subsystem1/53(VIPAll2RHMIRclReq)
  HMIMode8RclReq_2L_Val_read/1 -> Subsystem1/54(Lug2LHMIRclReq)
  HMIMode9RclReq_2R_Val_read/1 -> Subsystem1/55(Lug2RHMIRclReq)
  HMIMode3RclReq_2L_Val_read/1 -> Subsystem1/56(LugAll2LHMIRclReq)
  HMIMode3RclReq_2R_Val_read/1 -> Subsystem1/57(LugAll2RHMIRclReq)
  StSrvReq_Md2_Val_read/1 -> Subsystem1/58(StPassVipAllReq)
  StSrvReq_Md3_Val_read/1 -> Subsystem1/59(StPassLugAllReq)
  StSrvReq_Md5_Val_read/1 -> Subsystem1/60(StPassIntimacyLtMdReq)
  StSrvReq_Md20_Val_read/1 -> Subsystem1/61(StPassIntimacyRtMdReq)
  HMIMode5RclReq_2L_Val_read/1 -> Subsystem1/62(IntimacyLMdHMI2LRclReq)
  HMIMode20RclReq_2R_Val_read/1 -> Subsystem1/63(IntimacyRMdHMI2RRclReq)
  IntimacyLMdAvl_Val_read/1 -> Subsystem1/64(IntimacyLMdAvl)
  IntimacyRMdAvl_Val_read/1 -> Subsystem1/65(IntimacyRMdAvl)
  StSrvReq_Md7_Val_read/1 -> Subsystem1/66(StPassFamilyMdLtReq)
  HMIMode7RclReq_2L_Val_read/1 -> Subsystem1/67(FamilyMdHMI2LRclReq)
  HMIMode6RclReq_2R_Val_read/1 -> Subsystem1/68(FamilyMdHMI2RRclReq)
  FamilyMdLtAvl_Val_read/1 -> Subsystem1/69(FamilyMdLtAvl)
  FamilyMdRtAvl_Val_read/1 -> Subsystem1/71(FamilyMdRtAvl)
  StSrvReq_Md6_Val_read/1 -> Subsystem1/70(PassFamilyMdRtReq)
  StSrvReq_Md14_Val_read/1 -> Subsystem1/72(PassLyingMdLtReq)
  StSrvReq_Md15_Val_read/1 -> Subsystem1/73(PassLyingMdRtReq)
  HMIMode14RclReq_2L_Val_read/1 -> Subsystem1/74(LyingMdHMI2LRclReq)
  HMIMode15RclReq_2R_Val_read/1 -> Subsystem1/75(LyingMdHMI2RRclReq)
  LyingMdLtAvl_Val_read/1 -> Subsystem1/76(LyingMdLtAvl)
  LyingMdRtAvl_Val_read/1 -> Subsystem1/77(LyingMdRtAvl)
  AcsEntrySwValid_Val_read/1 -> Subsystem1/78(AcsEntrySwValid)
  VipRcvySwValid_Val_read/1 -> Subsystem1/79(VipRcvySwValid)
  StSrvReq_Md16_Val_read/1 -> Subsystem1/80(PassLgrstOpenLtMdReq)
  StSrvReq_Md17_Val_read/1 -> Subsystem1/81(PassLgrstCloseLtMdReq)
  LgrstOpenLtMdAvl_Val_read/1 -> Subsystem1/82(LgrstOpenLtMdAvl)
  LgrstOpenRtMdAvl_Val_read/1 -> Subsystem1/88(LgrstOpenRtMdAvl)
  LgrstCloseLtMdAvl_Val_read/1 -> Subsystem1/83(LgrstCloseLtMdAvl)
  LgrstCloseRtMdAvl_Val_read/1 -> Subsystem1/89(LgrstCloseRtMdAvl)
  HMIMode16RclReq_2L_Val_read/1 -> Subsystem1/84(LgrstOpenLtMdHMI2LRclReq)
  HMIMode17RclReq_2L_Val_read/1 -> Subsystem1/85(LgrstCloseLtMdHMI2LRclReq)
  StSrvReq_Md18_Val_read/1 -> Subsystem1/86(PassLgrstOpenRtMdReq)
  StSrvReq_Md19_Val_read/1 -> Subsystem1/87(PassLgrstCloseRtMdReq)
  HMIMode18RclReq_2R_Val_read/1 -> Subsystem1/90(LgrstOpenRtMdHMI2RRclReq)
  HMIMode19RclReq_2R_Val_read/1 -> Subsystem1/91(LgrstCloseRtMdHMI2RRclReq)
  SRSSlctSwReq_Val_read/1 -> Subsystem1/92(SRSSlctSwReq)
  Subsystem1/103(MdSWIntSrc) -> MdSWIntSrc_Val_write/1
  AcsEntry4s2LAvl_Val_read/1 -> Subsystem1/93(AcsEntry4s2LAvl)
  EZE4SSwReq_Val_read/1 -> Subsystem1/94(EZE4SSwReq)
  HMIMode21RclReq_2L_Val_read/1 -> Subsystem1/95(HMIMode21RclReq_2L)
  StSrvReq_Md21_Val_read/1 -> Subsystem1/96(PassAcsEntry4s2LReq)
  Subsystem1/104(acsEntry4s2LReq) -> acsEntry4s2LReq_Val_write/1
  Subsystem1/105(acsEntry4s2LSoftInt) -> acsEntry4s2LSoftInt_Val_write/1
  Subsystem1/106(acsEntry4s2LSrcTp) -> acsEntry4s2LSrcTp_Val_write/1
  Subsystem1/107(SwAcsEntry4s2LIntCnt) -> SwAcsEntry4s2LIntCnt_Val_write/1
  Subsystem1/108(AcsEntry4s2LNotf1ChimeEventStat) -> AcsEntry4s2LNotf1ChimeEventStat_Val_write/1
  AcsExit4s2LAvl_Val_read/1 -> Subsystem1/97(AcsExit4s2LAvl)
  HMIMode22RclReq_2L_Val_read/1 -> Subsystem1/98(HMIMode22RclReq_2L)
  StSrvReq_Md22_Val_read/1 -> Subsystem1/99(PassAcsExit4s2LReq)
  Subsystem1/110(acsExit4s2LReq) -> acsExit4s2LReq_Val_write/1
  Subsystem1/111(acsExit4s2LSoftInt) -> acsExit4s2LSoftInt_Val_write/1
  Subsystem1/112(SwAcsExit4s2LIntCnt) -> SwAcsExit4s2LIntCnt_Val_write/1
  Subsystem1/113(AcsExit4s2LNotf1ChimeEventStat) -> AcsExit4s2LNotf1ChimeEventStat_Val_write/1
  Subsystem1/114(acsExit4s2LSrcTp) -> acsExit4s2LSrcTp_Val_write/1
  AcsEntry4s2RAvl_Val_read/1 -> Subsystem1/100(AcsEntry4s2RAvl)
  HMIMode23RclReq_2R_Val_read/1 -> Subsystem1/101(HMIMode23RclReq_2R)
  StSrvReq_Md23_Val_read/1 -> Subsystem1/102(PassAcsEntry4s2RReq)
  Subsystem1/117(acsEntry4s2RReq) -> acsEntry4s2RReq_Val_write/1
  Subsystem1/118(acsEntry4s2RSoftInt) -> acsEntry4s2RSoftInt_Val_write/1
  Subsystem1/119(AcsEntry4s2RNotf1ChimeEventStat) -> AcsEntry4s2RNotf1ChimeEventStat_Val_write/1
  Subsystem1/116(SwAcsEntry4s2RIntCnt) -> SwAcsEntry4s2RIntCnt_Val_write/1
  Subsystem1/120(acsEntry4s2RSrcTp) -> acsEntry4s2RSrcTp_Val_write/1
  AcsExit4s2RAvl_Val_read/1 -> Subsystem1/103(AcsExit4s2RAvl)
  AcsMdExt4SSwRtRclReq_Val_read/1 -> Subsystem1/104(AcsMdExt4SSwRtRclReq)
  AcsMdExt4SSwRtRclReqV_Val_read/1 -> Subsystem1/105(AcsMdExt4SSwRtRclReqV)
  HMIMode24RclReq_2R_Val_read/1 -> Subsystem1/106(HMIMode24RclReq_2R)
  StSrvReq_Md24_Val_read/1 -> Subsystem1/107(PassAcsExit4s2RReq)
  Subsystem1/122(acsExit4s2RSoftInt) -> acsExit4s2RSoftInt_Val_write/1
  Subsystem1/123(acsExit4s2RReq) -> acsExit4s2RReq_Val_write/1
  Subsystem1/124(AcsExit4s2RNotf1ChimeEventStat) -> AcsExit4s2RNotf1ChimeEventStat_Val_write/1
  Subsystem1/125(SwAcsExit4s2RIntCnt) -> SwAcsExit4s2RIntCnt_Val_write/1
  Subsystem1/126(acsExit4s2RSrcTp) -> acsExit4s2RSrcTp_Val_write/1
  Subsystem1/127(SRSAcsExit4s2RIntCnt) -> SRSAcsExit4s2RIntCnt_Val_write/1
  Subsystem1/121(SRSAcsEntry4s2RIntCnt) -> SRSAcsEntry4s2RIntCnt_Val_write/1
  Subsystem1/115(SRSAcsExit4s2LIntCnt) -> SRSAcsExit4s2LIntCnt_Val_write/1
  Subsystem1/109(SRSAcsEntry4s2LIntCnt) -> SRSAcsEntry4s2LIntCnt_Val_write/1
  AcsEntryAll4sFwdAvl_Val_read/1 -> Subsystem1/114(AcsEntryAll4sFwdAvl)
  LckUlckActvtFunc_Val_read/1 -> Subsystem1/108(LckUlckActvtFunc)
  NotSecRowLeSeaOccStat_Val_read/1 -> Subsystem1/109(NotSecRowLeSeaOccStat)
  NotSecRowRtSeaOccStat_Val_read/1 -> Subsystem1/110(NotSecRowRtSeaOccStat)
  SysPwrMd_Val_read/1 -> Subsystem1/111(SysPwrMd)
  SysPwrMdV_Val_read/1 -> Subsystem1/112(SysPwrMdV)
  VehMovState_Val_read/1 -> Subsystem1/113(VehMovState)
  Subsystem1/130(AcsEntryAll4sFwdNotf1ChimeEventStat) -> AcsEntryAll4sFwdNotf1ChimeEventStat_Val_write/1
  Subsystem1/128(acsEntryAll4sFwdReq) -> acsEntryAll4sFwdReq_Val_write/1
  Subsystem1/129(acsEntryAll4sFwdSoftInt) -> acsEntryAll4sFwdSoftInt_Val_write/1
  LstLckChange_Val_read/1 -> Subsystem1/116(LstLckChange)
  LstLckFunc_Val_read/1 -> Subsystem1/115(LstLckFunc)
  RLDoorAjarSwAct_Val_read/1 -> Subsystem1/117(RLDoorAjarSwAct)
  RRDoorAjarSwAct_Val_read/1 -> Subsystem1/118(RRDoorAjarSwAct)
  PA_KeSMSwSeatSMSSeatMdTrigGapTimer_Val/1 -> Subsystem1/119(KeSMSwSeatSMSSeatMdTrigGapTimer)
  AcsEntryAll4sBwdAvl_Val_read/1 -> Subsystem1/120(AcsEntryAll4sBwdAvl)
  Subsystem1/131(acsEntryAll4sBwdReq) -> acsEntryAll4sBwdReq_Val_write/1
  Subsystem1/132(acsEntryAll4sBwdSoftInt) -> acsEntryAll4sBwdSoftInt_Val_write/1
  Subsystem1/133(acsEntryAll4sBwdNotf1ChimeEventStat) -> AcsEntryAll4sBwdNotf1ChimeEventStat_Val_write/1
  IfVeSMSeStNumConfig_Val_read/1 -> Subsystem1/121(IfVeSMSeStNumConfig_Val_read)
  Subsystem1/134(acsEntryAll4sFwdReqSig) -> acsEntryAll4sFwdReqSig_Val_write/1
  Subsystem1/135(acsEntryAll4sBwdReqSig) -> acsEntryAll4sBwdReqSig_Val_write/1
  PA_KeSMSwSeatTrigWaitTimer_Val/1 -> Subsystem1/122(KeSMSwSeatTrigWaitTimer)
  PasReclinerAvl_Val_read/1 -> Subsystem1/123(PasReclinerAvl)
  PassStFldDnMovSwAct_Val_read/1 -> Subsystem1/124(PassStFldDnMovSwAct)
  PassStFldDnMovSwActV_Val_read/1 -> Subsystem1/125(PassStFldDnMovSwActV)
  PassStFldUpMovSwAct_Val_read/1 -> Subsystem1/126(PassStFldUpMovSwAct)
  PassStFldUpMovSwActV_Val_read/1 -> Subsystem1/127(PassStFldUpMovSwActV)
  StSrvReq_Md30_Val_read/1 -> Subsystem1/128(StPassPasReclinerEntryReq)
  StSrvReq_Md31_Val_read/1 -> Subsystem1/129(StPassPasReclinerExitReq)
  ThdRLtStExpdSwReq_Val_read/1 -> Subsystem1/130(ThdRLtStExpdSwReq)
  ThdRLtStExpdSwReqV_Val_read/1 -> Subsystem1/131(ThdRLtStExpdSwReqV)
  ThdRRtStExpdSwReq_Val_read/1 -> Subsystem1/132(ThdRRtStExpdSwReq)
  ThdRRtStExpdSwReqV_Val_read/1 -> Subsystem1/133(ThdRRtStExpdSwReqV)
  PA_KeSMSuFoldType_Val/1 -> Subsystem1/134(KeSMSuFoldType)
  unfold3LAvl_Val_read/1 -> Subsystem1/135(unfold3LAvl)
  unfold3RAvl_Val_read/1 -> Subsystem1/136(unfold3RAvl)
  VipLtOutMdAvl_Val_read/1 -> Subsystem1/137(VipLtOutMdAvl)
  VipRtOutMdAvl_Val_read/1 -> Subsystem1/138(VipRtOutMdAvl)
  StSrvReq_Md27_Val_read/1 -> Subsystem1/139(StPassVIPLtOutReq)
  StSrvReq_Md28_Val_read/1 -> Subsystem1/140(StPassVIPRtOutReq)
  StSrvReq_Md29_Val_read/1 -> Subsystem1/141(StPassVIPAllOutReq)
  Subsystem1/148(Unfold3LReq) -> Unfold3LReq_Val_write/1
  Subsystem1/137(PasReclinerEntryReq) -> PasReclinerEntryReq_Val_write/1
  Subsystem1/138(PasReclinerEntrySrcReqTp) -> PasReclinerEntrySrcReqTp_Val_write/1
  Subsystem1/139(PasReclinerEntrySoftInt) -> PasReclinerEntrySoftInt_Val_write/1
  Subsystem1/140(PasReclinerEntryNotf1ChimeEventStat) -> PasReclinerEntryNotf1ChimeEventStat_Val_write/1
  Subsystem1/142(PasReclinerExitReq) -> PasReclinerExitReq_Val_write/1
  Subsystem1/143(PasReclinerExitSrcReqTp) -> PasReclinerExitSrcReqTp_Val_write/1
  Subsystem1/144(PasReclinerExitSoftInt) -> PasReclinerExitSoftInt_Val_write/1
  Subsystem1/145(PasReclinerExitNotf1ChimeEventStat) -> PasReclinerExitNotf1ChimeEventStat_Val_write/1
  Subsystem1/149(Unfold3LsrcReqTp) -> Unfold3LsrcReqTp_Val_write/1
  Subsystem1/150(Unfold3LNotf1ChimeEventStat) -> Unfold3LNotf1ChimeEventStat_Val_write/1
  Subsystem1/151(Unfold3RReq) -> Unfold3RReq_Val_write/1
  Subsystem1/152(Unfold3RsrcReqTp) -> Unfold3RsrcReqTp_Val_write/1
  Subsystem1/153(Unfold3RNotf1ChimeEventStat) -> Unfold3RNotf1ChimeEventStat_Val_write/1
  Subsystem1/154(VIPLtOutReq) -> VIPLtOutReq_Val_write/1
  Subsystem1/155(VIPLtOutsrcReqTp) -> VIPLtOutsrcReqTp_Val_write/1
  Subsystem1/156(VIPLtOutSoftInt) -> VIPLtOutSoftInt_Val_write/1
  Subsystem1/157(VIPLtOutNotf1ChimeEventStat) -> VIPLtOutNotf1ChimeEventStat_Val_write/1
  Subsystem1/158(VIPRtOutReq) -> VIPRtOutReq_Val_write/1
  Subsystem1/159(VIPRtOutsrcReqTp) -> VIPRtOutsrcReqTp_Val_write/1
  Subsystem1/160(VIPRtOutSoftInt) -> VIPRtOutSoftInt_Val_write/1
  Subsystem1/161(VIPRtOutNotf1ChimeEventStat) -> VIPRtOutNotf1ChimeEventStat_Val_write/1
  Subsystem1/162(VIPAllOutReq) -> VIPAllOutReq_Val_write/1
  Subsystem1/163(VIPAllOutsrcReqTp) -> VIPAllOutsrcReqTp_Val_write/1
  Subsystem1/164(VIPAllOutSoftInt) -> VIPAllOutSoftInt_Val_write/1
  Subsystem1/165(VIPAllOutNotf1ChimeEventStat) -> VIPAllOutNotf1ChimeEventStat_Val_write/1
  Subsystem1/146(SwUnfold3LIntCnt) -> SwUnfold3LIntCnt_Val_write/1
  Subsystem1/147(SwUnfold3RIntCnt) -> SwUnfold3RIntCnt_Val_write/1
  Subsystem1/141(SwPasReclinerExitIntCnt) -> SwPasReclinerExitIntCnt_Val_write/1
  Subsystem1/136(SwPasReclinerEntryIntCnt) -> SwPasReclinerEntryIntCnt_Val_write/1
  PasReclinerExitAvl_Val_read/1 -> Subsystem1/142(PasReclinerExitAvl)
  StPassCmprtMdHMIReqExt2_Val_read/1 -> Subsystem1/143(StPassCmprtMdHMIReqExt2)
  StSrvReq_Md32_Val_read/1 -> Subsystem1/144(StPassUnfold3LReq)
  Subsystem1/166(Big4SeatNotf1ChimeEventStat) -> Big4SeatNotf1ChimeEventStat_Val_write/1
  Subsystem1/167(Big4SeatReq) -> Big4SeatReq_Val_write/1
  Subsystem1/168(Big4SeatSoftInt) -> Big4SeatSoftInt_Val_write/1
  Subsystem1/169(Big4SeatsrcReqTp) -> Big4SeatsrcReqTp_Val_write/1
  Subsystem1/170(Unfold3LSoftInt) -> Unfold3LSoftInt_Val_write/1
  Subsystem1/171(Unfold3RSoftInt) -> Unfold3RSoftInt_Val_write/1
  Subsystem1/172("ExVIPRReq ") -> ExVIPRReq_Val_write/1
  Subsystem1/173(ExVIPRsrcReqTp) -> ExVIPRsrcReqTp_Val_write/1
  Subsystem1/174(ExVIPRSoftInt) -> ExVIPRSoftInt_Val_write/1
  Subsystem1/175(ExVIPRNotf1ChimeEventStat) -> ExVIPRNotf1ChimeEventStat_Val_write/1
  Subsystem1/176(ExVIPROutReq) -> ExVIPROutReq_Val_write/1
  Subsystem1/177(ExVIPROutsrcReqTp) -> ExVIPROutsrcReqTp_Val_write/1
  Subsystem1/178(ExVIPROutSoftInt) -> ExVIPROutSoftInt_Val_write/1
  Subsystem1/179(ExVIPROutNotf1ChimeEventStat) -> ExVIPROutNotf1ChimeEventStat_Val_write/1
  Big4SeatAvl_Val_read/1 -> Subsystem1/145(Big4SeatAvl)
  M61WholeVehMemAvl_Val_read/1 -> Subsystem1/146(M61WholeVehMemAvl)
  M62WholeVehMemAvl_Val_read/1 -> Subsystem1/147(M62WholeVehMemAvl)
  Subsystem1/180(WholeVehMem1Req) -> WholeVehMem1Req_Val_write/1
  Subsystem1/181(WholeVehMem1Notf1ChimeEventStat) -> WholeVehMem1Notf1ChimeEventStat_Val_write/1
  Subsystem1/182(WholeVehMem1SoftInt) -> WholeVehMem1SoftInt_Val_write/1
  Subsystem1/183(WholeVehMem1srcReqTp) -> WholeVehMem1srcReqTp_Val_write/1
  Subsystem1/184(WholeVehMem2Notf1ChimeEventStat) -> WholeVehMem2Notf1ChimeEventStat_Val_write/1
  Subsystem1/185(WholeVehMem2Req) -> WholeVehMem2Req_Val_write/1
  Subsystem1/186(WholeVehMem2SoftInt) -> WholeVehMem2SoftInt_Val_write/1
  Subsystem1/187(WholeVehMem2srcReqTp) -> WholeVehMem2srcReqTp_Val_write/1
  PA_StPassCmprtMdCtrl_Md1_VCUConfig_Val/1 -> Subsystem1/148(StPassCmprtMdCtrl_Md1_VCUConfig)
  PA_StPassCmprtMdCtrl_Md10_VCUConfig_Val/1 -> Subsystem1/149(StPassCmprtMdCtrl_Md10_VCUConfig)
  PA_StPassCmprtMdCtrl_Md11_VCUConfig_Val/1 -> Subsystem1/150(StPassCmprtMdCtrl_Md11_VCUConfig)
  PA_StPassCmprtMdCtrl_Md12_VCUConfig_Val/1 -> Subsystem1/151(StPassCmprtMdCtrl_Md12_VCUConfig)
  PA_StPassCmprtMdCtrl_Md13_VCUConfig_Val/1 -> Subsystem1/152(StPassCmprtMdCtrl_Md13_VCUConfig)
  PA_StPassCmprtMdCtrl_Md2_VCUConfig_Val/1 -> Subsystem1/153(StPassCmprtMdCtrl_Md2_VCUConfig)
  PA_StPassCmprtMdCtrl_Md27_VCUConfig_Val/1 -> Subsystem1/154(StPassCmprtMdCtrl_Md27_VCUConfig)
  PA_StPassCmprtMdCtrl_Md28_VCUConfig_Val/1 -> Subsystem1/155(StPassCmprtMdCtrl_Md28_VCUConfig)
  PA_StPassCmprtMdCtrl_Md29_VCUConfig_Val/1 -> Subsystem1/156(StPassCmprtMdCtrl_Md29_VCUConfig)
  PA_StPassCmprtMdCtrl_Md3_VCUConfig_Val/1 -> Subsystem1/157(StPassCmprtMdCtrl_Md3_VCUConfig)
  PA_StPassCmprtMdCtrl_Md30_VCUConfig_Val/1 -> Subsystem1/158(StPassCmprtMdCtrl_Md30_VCUConfig)
  PA_StPassCmprtMdCtrl_Md31_VCUConfig_Val/1 -> Subsystem1/159(StPassCmprtMdCtrl_Md31_VCUConfig)
  PA_StPassCmprtMdCtrl_Md32_VCUConfig_Val/1 -> Subsystem1/160(StPassCmprtMdCtrl_Md32_VCUConfig)
  PA_StPassCmprtMdCtrl_Md53_VCUConfig_Val/1 -> Subsystem1/161(StPassCmprtMdCtrl_Md53_VCUConfig)
  PA_StPassCmprtMdCtrl_Md56_VCUConfig_Val/1 -> Subsystem1/162(StPassCmprtMdCtrl_Md56_VCUConfig)
  PA_StPassCmprtMdCtrl_Md57_VCUConfig_Val/1 -> Subsystem1/163(StPassCmprtMdCtrl_Md57_VCUConfig)
  PA_StPassCmprtMdCtrl_Md58_VCUConfig_Val/1 -> Subsystem1/164(StPassCmprtMdCtrl_Md58_VCUConfig)
  PA_StPassCmprtMdCtrl_Md61_VCUConfig_Val/1 -> Subsystem1/165(StPassCmprtMdCtrl_Md61_VCUConfig)
  PA_StPassCmprtMdCtrl_Md62_VCUConfig_Val/1 -> Subsystem1/166(StPassCmprtMdCtrl_Md62_VCUConfig)
  PA_StPassCmprtMdCtrl_Md8_VCUConfig_Val/1 -> Subsystem1/167(StPassCmprtMdCtrl_Md8_VCUConfig)
  PA_StPassCmprtMdCtrl_Md9_VCUConfig_Val/1 -> Subsystem1/168(StPassCmprtMdCtrl_Md9_VCUConfig)
  PA_StSrv_StMd1_Config_Val/1 -> Subsystem1/169(StSrv_StMd1_Config)
  PA_StSrv_StMd10_Config_Val/1 -> Subsystem1/170(StSrv_StMd10_Config)
  PA_StSrv_StMd11_Config_Val/1 -> Subsystem1/171(StSrv_StMd11_Config)
  PA_StSrv_StMd12_Config_Val/1 -> Subsystem1/172(StSrv_StMd12_Config)
  PA_StSrv_StMd13_Config_Val/1 -> Subsystem1/173(StSrv_StMd13_Config)
  PA_StSrv_StMd2_Config_Val/1 -> Subsystem1/174(StSrv_StMd2_Config)
  PA_StSrv_StMd27_Config_Val/1 -> Subsystem1/175(StSrv_StMd27_Config)
  PA_StSrv_StMd28_Config_Val/1 -> Subsystem1/176(StSrv_StMd28_Config)
  PA_StSrv_StMd29_Config_Val/1 -> Subsystem1/177(StSrv_StMd29_Config)
  PA_StSrv_StMd3_Config_Val/1 -> Subsystem1/178(StSrv_StMd3_Config)
  PA_StSrv_StMd30_Config_Val/1 -> Subsystem1/179(StSrv_StMd30_Config)
  PA_StSrv_StMd31_Config_Val/1 -> Subsystem1/180(StSrv_StMd31_Config)
  PA_StSrv_StMd32_Config_Val/1 -> Subsystem1/181(StSrv_StMd32_Config)
  PA_StSrv_StMd8_Config_Val/1 -> Subsystem1/182(StSrv_StMd8_Config)
  PA_StSrv_StMd9_Config_Val/1 -> Subsystem1/183(StSrv_StMd9_Config)
